simulink library "lib_Lagrangian_Model_Nonlinear_R2012a"  (Simulink 7.9)
settings: Solver=ode45  StartTime=0.0  StopTime=10.0  RelTol=1e-3
undefined symbols (not defined in the file): TRMS
settings Model: Creator=ottoe  LastModifiedBy=ottoe  CovModelRefEnable=off

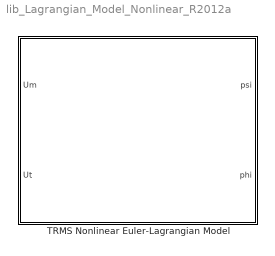
== system lib_Lagrangian_Model_Nonlinear_R2012a ==
  TRMS Nonlinear Euler-Lagrangian Model : Subsystem  mask(Physical model){Psi_zero=0, Psi_dot_zero=0, Phi_zero=0, Phi_dot_zero=0, Wm_zero=0, Wt_zero=0}
      mask prompts: Psi_zero "Psi"; Psi_dot_zero "Psi_dot"; Phi_zero "Phi"; Phi_dot_zero "Phi_dot"; Wm_zero "Wm"; Wt_zero "Wt"
      mask help:
      | Nonlinear mathematical model of the TRMS based on the Euler-Lagrangian approach.
      |
      | References:
      | RAO, Vidya S; BHAT, Akhila; MORALES-VIVIESCAS, Rafael M. Extended Kalman observer based Robust Control of one degree of freedom TRMS. Proceedings of the 12th Asian Control Conference (ASCC). Kitakyushu, Japan, June 9-12, 2019.
      |
      | TASTEMIROV, Azamat; LECCHINI-VISINTINI, Andrea; MORALES-VIVIESCAS, Rafael M. Complete dynamic model of the Twin Rotor MIMO System (TRMS) with experimental validation. Control Engineering Practice, vol. 66, pp. 89-98 (2017).
      mask Display: image(imread('TRMS.jpg'));

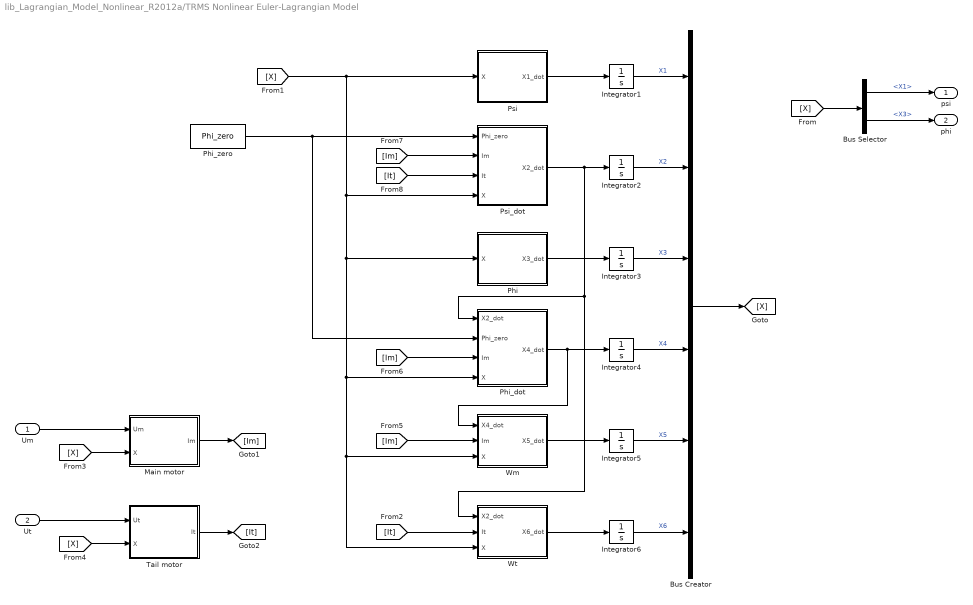
== system lib_Lagrangian_Model_Nonlinear_R2012a/TRMS Nonlinear Euler-Lagrangian Model ==
  Um : Inport
  Ut : Inport  Port=2
  Bus Creator : BusCreator  Inputs=6
  Bus Selector : BusSelector  OutputSignals=X1,X3
  Integrator1 : Integrator  InitialCondition=Psi_zero  ContinuousStateAttributes='Psi'
  Integrator2 : Integrator  InitialCondition=Psi_dot_zero  ContinuousStateAttributes='Psi_dot'
  Integrator3 : Integrator  InitialCondition=Phi_zero  ContinuousStateAttributes='Phi'
  Integrator4 : Integrator  InitialCondition=Phi_dot_zero  ContinuousStateAttributes='Phi_dot'
  Integrator5 : Integrator  InitialCondition=Wm_zero  ContinuousStateAttributes='Wm'
  Integrator6 : Integrator  InitialCondition=Wt_zero  ContinuousStateAttributes='Wt'
  Main motor : Subsystem
  Phi : Subsystem
  Phi_dot : Subsystem
  Phi_zero : Constant  Value=Phi_zero
  Psi : Subsystem
  Psi_dot : Subsystem
  Tail motor : Subsystem
  Wm : Subsystem
  Wt : Subsystem
  psi : Outport
  phi : Outport  Port=2
  wires:
  Bus Selector/1 -> psi/1  "<X1>"
  Wm/1(X5_dot) -> Integrator5/1
  Integrator5/1 -> Bus Creator/5  "X5"
  Psi/1(X1_dot) -> Integrator1/1
  [X] -> Tail motor/2(X)
  Ut/1 -> Tail motor/1(Ut)
  Um/1 -> Main motor/1(Um)
  [X] -> Main motor/2(X)
  Wt/1(X6_dot) -> Integrator6/1
  [X] -> Bus Selector/1
  Bus Selector/2 -> phi/1  "<X3>"
  Integrator4/1 -> Bus Creator/4  "X4"
  Phi_dot/1(X4_dot) -> Wm/1(X4_dot), Integrator4/1
  Integrator1/1 -> Bus Creator/1  "X1"
  Integrator2/1 -> Bus Creator/2  "X2"
  Bus Creator/1 -> [X]
  Integrator3/1 -> Bus Creator/3  "X3"
  Integrator6/1 -> Bus Creator/6  "X6"
  [X] -> Psi/1(X), Phi/1(X), Wt/3(X), Wm/3(X), Phi_dot/4(X), Psi_dot/4(X)
  Main motor/1(Im) -> [Im]
  Tail motor/1(It) -> [It]
  [It] -> Wt/2(It)
  [Im] -> Wm/2(Im)
  [Im] -> Phi_dot/3(Im)
  Phi_zero/1 -> Psi_dot/1(Phi_zero), Phi_dot/2(Phi_zero)
  Phi/1(X3_dot) -> Integrator3/1
  [Im] -> Psi_dot/2(Im)
  [It] -> Psi_dot/3(It)
  Psi_dot/1(X2_dot) -> Wt/1(X2_dot), Phi_dot/1(X2_dot), Integrator2/1

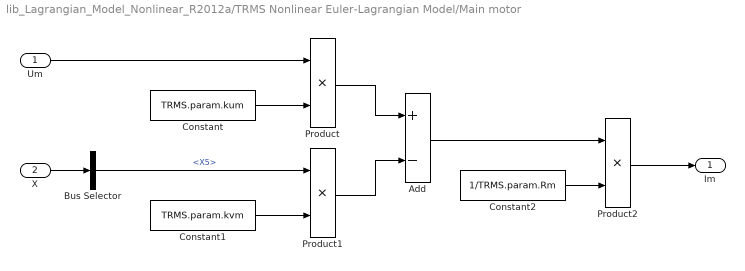
== system lib_Lagrangian_Model_Nonlinear_R2012a/TRMS Nonlinear Euler-Lagrangian Model/Main motor ==
  Um : Inport
  X : Inport  Port=2
  Add : Sum  Inputs=+-
  Bus Selector : BusSelector  OutputSignals=X5
  Constant : Constant  Value=TRMS.param.kum
  Constant1 : Constant  Value=TRMS.param.kvm
  Constant2 : Constant  Value=1/TRMS.param.Rm
  Product : Product
  Product1 : Product
  Product2 : Product
  Im : Outport
  wires:
  Um/1 -> Product/1
  Constant/1 -> Product/2
  Product/1 -> Add/1
  Constant1/1 -> Product1/2
  X/1 -> Bus Selector/1
  Product1/1 -> Add/2
  Bus Selector/1 -> Product1/1  "<X5>"
  Add/1 -> Product2/1
  Constant2/1 -> Product2/2
  Product2/1 -> Im/1

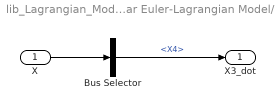
== system lib_Lagrangian_Model_Nonlinear_R2012a/TRMS Nonlinear Euler-Lagrangian Model/Phi ==
  X : Inport
  Bus Selector : BusSelector  OutputSignals=X4
  X3_dot : Outport
  wires:
  X/1 -> Bus Selector/1
  Bus Selector/1 -> X3_dot/1  "<X4>"

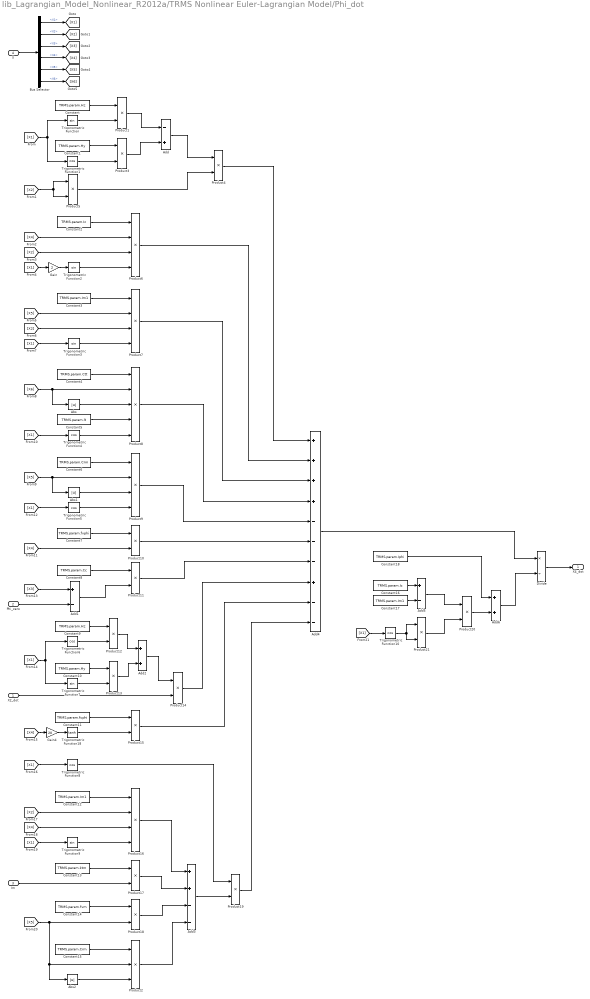
== system lib_Lagrangian_Model_Nonlinear_R2012a/TRMS Nonlinear Euler-Lagrangian Model/Phi_dot ==
  X2_dot : Inport
  Phi_zero : Inport  Port=2
  Im : Inport  Port=3
  X : Inport  Port=4
  Abs : Abs
  Abs1 : Abs
  Abs2 : Abs
  Add : Sum  Inputs=-+
  Add1 : Sum  Inputs=+-
  Add2 : Sum
  Add3 : Sum  Inputs=++--
  Add4 : Sum  Inputs=++++---+--
  Add5 : Sum  Inputs=+-
  Add6 : Sum
  Bus Selector : BusSelector  OutputSignals=X1,X2,X3,X4,X5,X6
  Constant : Constant  Value=TRMS.param.Hz
  Constant1 : Constant  Value=TRMS.param.Hy
  Constant10 : Constant  Value=TRMS.param.Hy
  Constant11 : Constant  Value=TRMS.param.fcphi
  Constant12 : Constant  Value=TRMS.param.Im1
  Constant13 : Constant  Value=TRMS.param.ktm
  Constant14 : Constant  Value=TRMS.param.fvm
  Constant15 : Constant  Value=TRMS.param.Crm
  Constant16 : Constant  Value=TRMS.param.Ic
  Constant17 : Constant  Value=TRMS.param.Im1
  Constant18 : Constant  Value=TRMS.param.Iphi
  Constant2 : Constant  Value=TRMS.param.Ic
  Constant3 : Constant  Value=TRMS.param.Im1
  Constant4 : Constant  Value=TRMS.param.Ctt
  Constant5 : Constant  Value=TRMS.param.lt
  Constant6 : Constant  Value=TRMS.param.Crm
  Constant7 : Constant  Value=TRMS.param.fvphi
  Constant8 : Constant  Value=TRMS.param.Cc
  Constant9 : Constant  Value=TRMS.param.Hz
  Divide : Product  Inputs=*/
  Gain : Gain  Gain=2
  Gain4 : Gain  Gain=20
  Product{1,3..5,10..15,17..21} (15 alike) : Product
  Product{6..7,9,16} (4 alike) : Product  Inputs=4
  Product2 : Product  Inputs=3
  Product8 : Product  Inputs=5
  Trigonometric Function{,2..3,7,9} (5 alike) : Trigonometry
  Trigonometric Function{1,4..6,8,10} (6 alike) : Trigonometry  Operator=cos
  Trigonometric Function18 : Trigonometry  Operator=tanh
  X4_dot : Outport
  wires:
  X/1 -> Bus Selector/1
  Bus Selector/1 -> [X1]  "<X1>"
  Bus Selector/2 -> [X2]  "<X2>"
  Bus Selector/3 -> [X3]  "<X3>"
  Bus Selector/4 -> [X4]  "<X4>"
  Bus Selector/5 -> [X5]  "<X5>"
  Bus Selector/6 -> [X6]  "<X6>"
  Constant/1 -> Product1/1
  Trigonometric Function/1 -> Product1/2
  Constant1/1 -> Product3/1
  Trigonometric Function1/1 -> Product3/2
  [X1] -> Trigonometric Function1/1, Trigonometric Function/1
  Product1/1 -> Add/1
  Product3/1 -> Add/2
  Add/1 -> Product4/1
  [X2] -> Product5/2, Product5/1
  Product5/1 -> Product4/2
  Constant2/1 -> Product6/1
  [X4] -> Product6/2
  [X2] -> Product6/3
  [X1] -> Gain/1
  Gain/1 -> Trigonometric Function2/1
  Trigonometric Function2/1 -> Product6/4
  Constant3/1 -> Product7/1
  [X5] -> Product7/2
  [X2] -> Product7/3
  [X1] -> Trigonometric Function3/1
  Trigonometric Function3/1 -> Product7/4
  [X1] -> Trigonometric Function4/1
  Constant4/1 -> Product8/1
  [X6] -> Abs/1, Product8/2
  Abs/1 -> Product8/3
  Constant5/1 -> Product8/4
  Trigonometric Function4/1 -> Product8/5
  Constant6/1 -> Product9/1
  [X5] -> Abs1/1, Product9/2
  [X1] -> Trigonometric Function5/1
  Trigonometric Function5/1 -> Product9/4
  Abs1/1 -> Product9/3
  Constant7/1 -> Product10/1
  [X4] -> Product10/2
  Constant8/1 -> Product11/1
  Add1/1 -> Product11/2
  [X3] -> Add1/1
  Phi_zero/1 -> Add1/2
  Constant9/1 -> Product12/1
  Trigonometric Function6/1 -> Product12/2
  Constant10/1 -> Product13/1
  Trigonometric Function7/1 -> Product13/2
  [X1] -> Trigonometric Function7/1, Trigonometric Function6/1
  Product12/1 -> Add2/1
  Product13/1 -> Add2/2
  Add2/1 -> Product14/1
  X2_dot/1 -> Product14/2
  Constant11/1 -> Product15/1
  Product17/1 -> Add3/2
  Product18/1 -> Add3/3
  Product16/1 -> Add3/1
  Product2/1 -> Add3/4
  [X1] -> Trigonometric Function8/1
  Constant12/1 -> Product16/1
  [X2] -> Product16/2
  [X4] -> Product16/3
  Trigonometric Function9/1 -> Product16/4
  [X1] -> Trigonometric Function9/1
  Constant13/1 -> Product17/1
  Im/1 -> Product17/2
  Constant14/1 -> Product18/1
  [X5] -> Abs2/1, Product2/2, Product18/2
  Constant15/1 -> Product2/1
  Abs2/1 -> Product2/3
  Product4/1 -> Add4/1
  Product6/1 -> Add4/2
  Product7/1 -> Add4/3
  Product8/1 -> Add4/4
  Product9/1 -> Add4/5
  Product10/1 -> Add4/6
  Product11/1 -> Add4/7
  Product14/1 -> Add4/8
  Product15/1 -> Add4/9
  Product19/1 -> Add4/10
  Add4/1 -> Divide/1
  Constant16/1 -> Add5/1
  Constant17/1 -> Add5/2
  Add5/1 -> Product20/1
  [X1] -> Trigonometric Function10/1
  Trigonometric Function10/1 -> Product21/2, Product21/1
  Product21/1 -> Product20/2
  Add6/1 -> Divide/2
  Divide/1 -> X4_dot/1
  Add3/1 -> Product19/2
  Trigonometric Function8/1 -> Product19/1
  Product20/1 -> Add6/2
  Constant18/1 -> Add6/1
  Gain4/1 -> Trigonometric Function18/1
  [X4] -> Gain4/1
  Trigonometric Function18/1 -> Product15/2

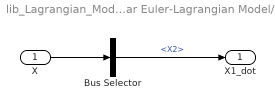
== system lib_Lagrangian_Model_Nonlinear_R2012a/TRMS Nonlinear Euler-Lagrangian Model/Psi ==
  X : Inport
  Bus Selector : BusSelector  OutputSignals=X2
  X1_dot : Outport
  wires:
  X/1 -> Bus Selector/1
  Bus Selector/1 -> X1_dot/1  "<X2>"

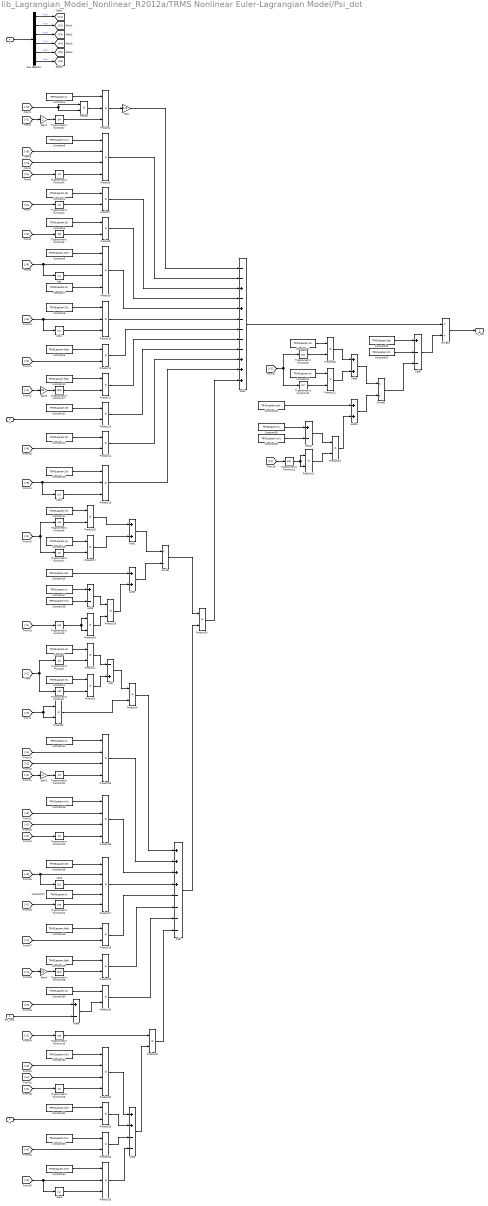
== system lib_Lagrangian_Model_Nonlinear_R2012a/TRMS Nonlinear Euler-Lagrangian Model/Psi_dot ==
  Phi_zero : Inport
  Im : Inport  Port=2
  It : Inport  Port=3
  X : Inport  Port=4
  Abs{,1..4} (5 alike) : Abs
  Add : Sum  Inputs=-+
  Add{1..2,6,10} (4 alike) : Sum
  Add11 : Sum  Inputs=+-
  Add3 : Sum  Inputs=+-
  Add4 : Sum  Inputs=--+-+----+++
  Add5 : Sum  Inputs=+--
  Add7 : Sum  Inputs=++++----
  Add8 : Sum  Inputs=+-
  Add9 : Sum  Inputs=++--
  Bus Selector : BusSelector  OutputSignals=X1,X2,X3,X4,X5,X6
  Constant : Constant  Value=TRMS.param.Hz
  Constant1 : Constant  Value=TRMS.param.Hy
  Constant10 : Constant  Value=TRMS.param.fcpsi
  Constant11 : Constant  Value=TRMS.param.ktt
  Constant12 : Constant  Value=TRMS.param.fvt
  Constant13 : Constant  Value=TRMS.param.Crt
  Constant14 : Constant  Value=TRMS.param.Hz
  Constant15 : Constant  Value=TRMS.param.Hy
  Constant16 : Constant  Value=TRMS.param.Iphi
  Constant{2,17,24,35} (4 alike) : Constant  Value=TRMS.param.Ic
  Constant{3,18,25,31,36} (5 alike) : Constant  Value=TRMS.param.Im1
  Constant19 : Constant  Value=TRMS.param.Ipsi
  Constant20 : Constant  Value=TRMS.param.It1
  Constant21 : Constant  Value=TRMS.param.Hz
  Constant22 : Constant  Value=TRMS.param.Hy
  Constant23 : Constant  Value=TRMS.param.Iphi
  Constant26 : Constant  Value=TRMS.param.Ctt
  Constant27 : Constant  Value=TRMS.param.lt
  Constant28 : Constant  Value=TRMS.param.fvphi
  Constant29 : Constant  Value=TRMS.param.fcphi
  Constant30 : Constant  Value=TRMS.param.Cc
  Constant32 : Constant  Value=TRMS.param.ktm
  Constant33 : Constant  Value=TRMS.param.fvm
  Constant34 : Constant  Value=TRMS.param.Crm
  Constant4 : Constant  Value=TRMS.param.Gz
  Constant5 : Constant  Value=TRMS.param.Gy
  Constant6 : Constant  Value=TRMS.param.Ctm
  Constant7 : Constant  Value=TRMS.param.lm
  Constant8 : Constant  Value=TRMS.param.Crt
  Constant9 : Constant  Value=TRMS.param.fvpsi
  Divide : Product  Inputs=*/
  Divide1 : Product  Inputs=*/
  Divide2 : Product  Inputs=*/
  Gain : Gain  Gain=1/2
  Gain1 : Gain  Gain=2
  Gain2 : Gain  Gain=2
  Gain3 : Gain  Gain=20
  Gain4 : Gain  Gain=20
  Product{,1,3..5,7..8,11..14,16..24,28..31,33..34} (26 alike) : Product
  Product{2,10,15,35} (4 alike) : Product  Inputs=3
  Product{6,9,25..26,32} (5 alike) : Product  Inputs=4
  Product27 : Product  Inputs=5
  Trigonometric Function{,2..4,7,10,12..13,16} (9 alike) : Trigonometry
  Trigonometric Function{1,5..6,8..9,11,14..15} (8 alike) : Trigonometry  Operator=cos
  Trigonometric Function17 : Trigonometry  Operator=tanh
  Trigonometric Function18 : Trigonometry  Operator=tanh
  X2_dot : Outport
  wires:
  Bus Selector/1 -> [X1]  "<X1>"
  Bus Selector/2 -> [X2]  "<X2>"
  Bus Selector/3 -> [X3]  "<X3>"
  Bus Selector/4 -> [X4]  "<X4>"
  Bus Selector/5 -> [X5]  "<X5>"
  Bus Selector/6 -> [X6]  "<X6>"
  Constant/1 -> Product1/1
  Trigonometric Function/1 -> Product1/2
  Constant1/1 -> Product3/1
  Trigonometric Function1/1 -> Product3/2
  [X1] -> Trigonometric Function1/1, Trigonometric Function/1
  Product1/1 -> Add/1
  Product3/1 -> Add/2
  Add/1 -> Product4/1
  [X2] -> Product5/2, Product5/1
  Product5/1 -> Product4/2
  X/1 -> Bus Selector/1
  [X1] -> Gain1/1
  Gain1/1 -> Trigonometric Function2/1
  Product2/1 -> Gain/1
  Constant2/1 -> Product2/1
  Trigonometric Function2/1 -> Product2/3
  Product/1 -> Product2/2
  [X4] -> Product/2, Product/1
  Constant3/1 -> Product6/1
  [X5] -> Product6/2
  [X4] -> Product6/3
  Trigonometric Function3/1 -> Product6/4
  [X1] -> Trigonometric Function3/1
  Constant4/1 -> Product7/1
  [X1] -> Trigonometric Function4/1
  Trigonometric Function4/1 -> Product7/2
  Constant5/1 -> Product8/1
  [X1] -> Trigonometric Function5/1
  Trigonometric Function5/1 -> Product8/2
  Constant6/1 -> Product9/1
  [X5] -> Abs/1, Product9/2
  Abs/1 -> Product9/3
  Constant7/1 -> Product9/4
  Constant8/1 -> Product10/1
  [X6] -> Product10/2, Abs1/1
  Abs1/1 -> Product10/3
  Constant9/1 -> Product11/1
  [X2] -> Product11/2
  Constant10/1 -> Product12/1
  Constant11/1 -> Product13/1
  Trigonometric Function17/1 -> Product12/2
  It/1 -> Product13/2
  Constant12/1 -> Product14/1
  [X6] -> Product14/2
  Constant13/1 -> Product15/1
  [X6] -> Product15/2, Abs2/1
  Abs2/1 -> Product15/3
  Constant14/1 -> Product16/1
  Trigonometric Function6/1 -> Product16/2
  Constant15/1 -> Product17/1
  Trigonometric Function7/1 -> Product17/2
  [X1] -> Trigonometric Function7/1, Trigonometric Function6/1
  Product16/1 -> Add1/1
  Product17/1 -> Add1/2
  Add1/1 -> Divide/1
  Add2/1 -> Divide/2
  Constant16/1 -> Add2/1
  [X1] -> Trigonometric Function8/1
  Trigonometric Function8/1 -> Product18/2, Product18/1
  Constant17/1 -> Add3/1
  Constant18/1 -> Add3/2
  Product19/1 -> Add2/2
  Divide/1 -> Product24/1
  Add7/1 -> Product24/2
  Product4/1 -> Add7/1
  Constant24/1 -> Product25/1
  [X4] -> Product25/2
  [X2] -> Product25/3
  [X1] -> Gain2/1
  Gain2/1 -> Trigonometric Function12/1
  Trigonometric Function12/1 -> Product25/4
  Product25/1 -> Add7/2
  Constant25/1 -> Product26/1
  [X5] -> Product26/2
  [X2] -> Product26/3
  [X1] -> Trigonometric Function13/1
  Trigonometric Function13/1 -> Product26/4
  Constant26/1 -> Product27/1
  [X6] -> Abs3/1, Product27/2
  Abs3/1 -> Product27/3
  Constant27/1 -> Product27/4
  [X1] -> Trigonometric Function14/1
  Trigonometric Function14/1 -> Product27/5
  Product26/1 -> Add7/3
  Product27/1 -> Add7/4
  Constant28/1 -> Product28/1
  [X4] -> Product28/2
  Product28/1 -> Add7/5
  Constant29/1 -> Product29/1
  Constant30/1 -> Product30/1
  Product29/1 -> Add7/6
  Add8/1 -> Product30/2
  [X3] -> Add8/1
  Phi_zero/1 -> Add8/2
  Product30/1 -> Add7/7
  [X1] -> Trigonometric Function15/1
  Trigonometric Function15/1 -> Product31/1
  Product31/1 -> Add7/8
  Add9/1 -> Product31/2
  Product33/1 -> Add9/2
  Product34/1 -> Add9/3
  Product35/1 -> Add9/4
  Product32/1 -> Add9/1
  Constant31/1 -> Product32/1
  [X2] -> Product32/2
  [X4] -> Product32/3
  [X1] -> Trigonometric Function16/1
  Trigonometric Function16/1 -> Product32/4
  Constant32/1 -> Product33/1
  Im/1 -> Product33/2
  Constant33/1 -> Product34/1
  [X5] -> Product34/2
  Constant34/1 -> Product35/1
  [X5] -> Abs4/1, Product35/2
  Abs4/1 -> Product35/3
  Gain/1 -> Add4/1
  Product6/1 -> Add4/2
  Product7/1 -> Add4/3
  Product8/1 -> Add4/4
  Product9/1 -> Add4/5
  Product10/1 -> Add4/6
  Product11/1 -> Add4/7
  Product12/1 -> Add4/8
  Product13/1 -> Add4/9
  Product14/1 -> Add4/10
  Product15/1 -> Add4/11
  Product24/1 -> Add4/12
  Add4/1 -> Divide1/1
  Divide1/1 -> X2_dot/1
  Add5/1 -> Divide1/2
  Constant19/1 -> Add5/1
  Constant20/1 -> Add5/2
  Add3/1 -> Product19/1
  Product18/1 -> Product19/2
  Constant21/1 -> Product20/1
  Trigonometric Function9/1 -> Product20/2
  Constant22/1 -> Product21/1
  Trigonometric Function10/1 -> Product21/2
  [X1] -> Trigonometric Function10/1, Trigonometric Function9/1
  Product20/1 -> Add6/1
  Product21/1 -> Add6/2
  Add6/1 -> Divide2/1
  Add10/1 -> Divide2/2
  Constant23/1 -> Add10/1
  [X1] -> Trigonometric Function11/1
  Trigonometric Function11/1 -> Product22/2, Product22/1
  Constant35/1 -> Add11/1
  Constant36/1 -> Add11/2
  Product23/1 -> Add10/2
  Add11/1 -> Product23/1
  Product22/1 -> Product23/2
  Divide2/1 -> Add5/3
  [X2] -> Gain3/1
  Gain3/1 -> Trigonometric Function17/1
  Gain4/1 -> Trigonometric Function18/1
  [X4] -> Gain4/1
  Trigonometric Function18/1 -> Product29/2

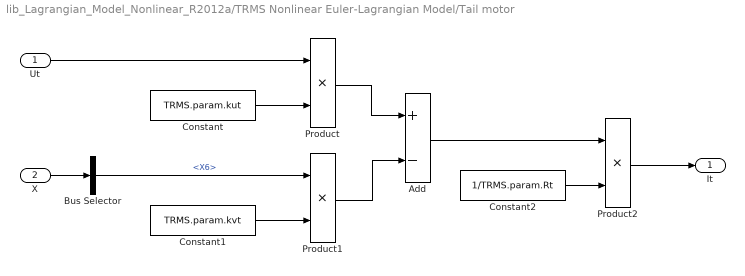
== system lib_Lagrangian_Model_Nonlinear_R2012a/TRMS Nonlinear Euler-Lagrangian Model/Tail motor ==
  Ut : Inport
  X : Inport  Port=2
  Add : Sum  Inputs=+-
  Bus Selector : BusSelector  OutputSignals=X6
  Constant : Constant  Value=TRMS.param.kut
  Constant1 : Constant  Value=TRMS.param.kvt
  Constant2 : Constant  Value=1/TRMS.param.Rt
  Product : Product
  Product1 : Product
  Product2 : Product
  It : Outport
  wires:
  X/1 -> Bus Selector/1
  Add/1 -> Product2/1
  Constant2/1 -> Product2/2
  Ut/1 -> Product/1
  Constant/1 -> Product/2
  Product/1 -> Add/1
  Bus Selector/1 -> Product1/1  "<X6>"
  Constant1/1 -> Product1/2
  Product1/1 -> Add/2
  Product2/1 -> It/1

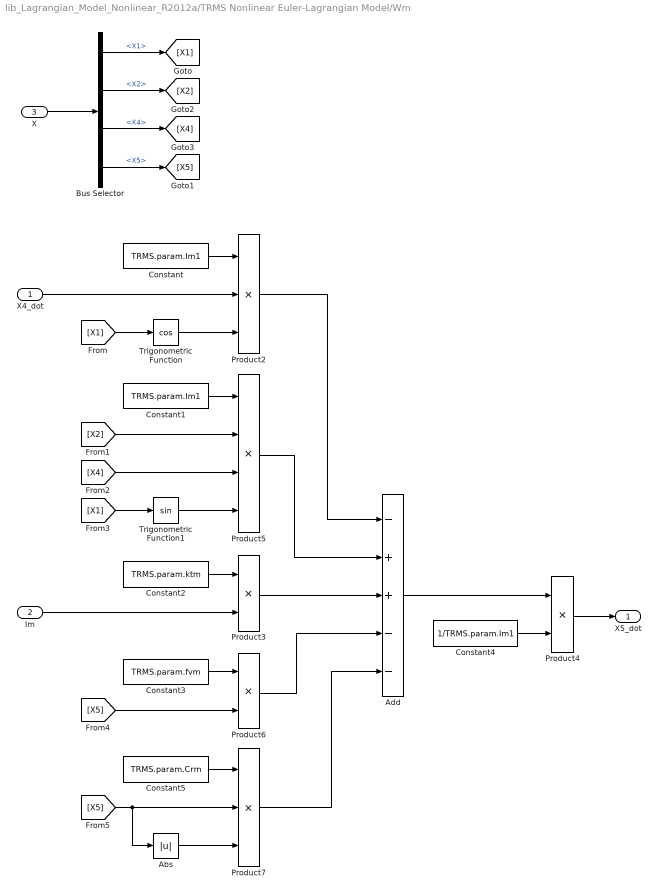
== system lib_Lagrangian_Model_Nonlinear_R2012a/TRMS Nonlinear Euler-Lagrangian Model/Wm ==
  X4_dot : Inport
  Im : Inport  Port=2
  X : Inport  Port=3
  Abs : Abs
  Add : Sum  Inputs=-++--
  Bus Selector : BusSelector  OutputSignals=X1,X2,X4,X5
  Constant : Constant  Value=TRMS.param.Im1
  Constant1 : Constant  Value=TRMS.param.Im1
  Constant2 : Constant  Value=TRMS.param.ktm
  Constant3 : Constant  Value=TRMS.param.fvm
  Constant4 : Constant  Value=1/TRMS.param.Im1
  Constant5 : Constant  Value=TRMS.param.Crm
  Product2 : Product  Inputs=3
  Product3 : Product
  Product4 : Product
  Product5 : Product  Inputs=4
  Product6 : Product
  Product7 : Product  Inputs=3
  Trigonometric Function : Trigonometry  Operator=cos
  Trigonometric Function1 : Trigonometry
  X5_dot : Outport
  wires:
  Constant4/1 -> Product4/2
  Add/1 -> Product4/1
  Product4/1 -> X5_dot/1
  X/1 -> Bus Selector/1
  Bus Selector/1 -> [X1]  "<X1>"
  Bus Selector/4 -> [X5]  "<X5>"
  [X1] -> Trigonometric Function/1
  Trigonometric Function/1 -> Product2/3
  Product2/1 -> Add/1
  Constant/1 -> Product2/1
  X4_dot/1 -> Product2/2
  Constant1/1 -> Product5/1
  Bus Selector/2 -> [X2]  "<X2>"
  Bus Selector/3 -> [X4]  "<X4>"
  [X2] -> Product5/2
  [X4] -> Product5/3
  [X1] -> Trigonometric Function1/1
  Trigonometric Function1/1 -> Product5/4
  Constant2/1 -> Product3/1
  Im/1 -> Product3/2
  Product5/1 -> Add/2
  Product3/1 -> Add/3
  Constant3/1 -> Product6/1
  [X5] -> Product6/2
  Product6/1 -> Add/4
  Constant5/1 -> Product7/1
  [X5] -> Abs/1, Product7/2
  Abs/1 -> Product7/3
  Product7/1 -> Add/5

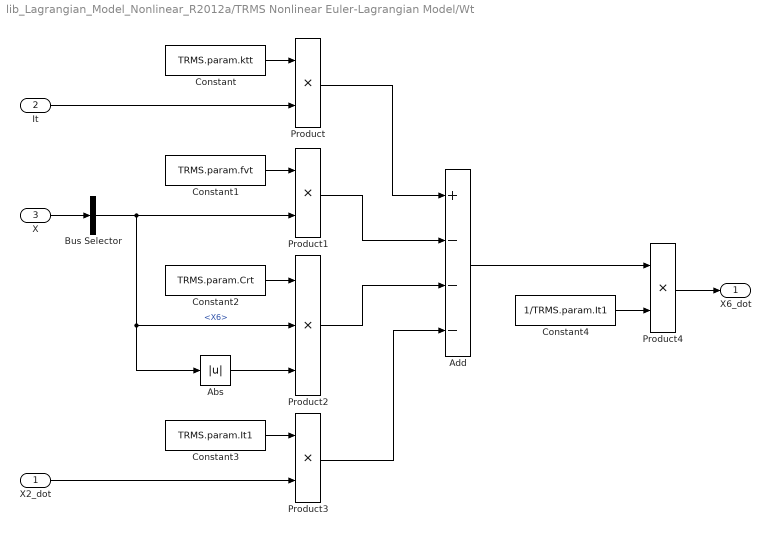
== system lib_Lagrangian_Model_Nonlinear_R2012a/TRMS Nonlinear Euler-Lagrangian Model/Wt ==
  X2_dot : Inport
  It : Inport  Port=2
  X : Inport  Port=3
  Abs : Abs
  Add : Sum  Inputs=+---
  Bus Selector : BusSelector  OutputSignals=X6
  Constant : Constant  Value=TRMS.param.ktt
  Constant1 : Constant  Value=TRMS.param.fvt
  Constant2 : Constant  Value=TRMS.param.Crt
  Constant3 : Constant  Value=TRMS.param.It1
  Constant4 : Constant  Value=1/TRMS.param.It1
  Product{,1,3..4} (4 alike) : Product
  Product2 : Product  Inputs=3
  X6_dot : Outport
  wires:
  Product/1 -> Add/1
  Product1/1 -> Add/2
  Product2/1 -> Add/3
  Product3/1 -> Add/4
  X/1 -> Bus Selector/1
  Bus Selector/1 -> Product1/2, Product2/2, Abs/1  "<X6>"
  Add/1 -> Product4/1
  Product4/1 -> X6_dot/1
  Constant4/1 -> Product4/2
  Constant/1 -> Product/1
  It/1 -> Product/2
  Constant1/1 -> Product1/1
  Constant2/1 -> Product2/1
  Abs/1 -> Product2/3
  Constant3/1 -> Product3/1
  X2_dot/1 -> Product3/2
